simulink model "Model_Mk2"  (R2024a)
settings: Solver=VariableStepAuto  StartTime=startTime  StopTime=stopTime  FixedStep=1e-4  RelTol=1e-9  AbsTol=1e-9  EnableMultiTasking=on
model workspace (MAT data in the model file):
  Kset = [-2.00916512617e-14 -2.1396164685e-13 1645.65145003 1.10700309911e-13 0.064606154931 -1.15620600709 -2.35613942722e-12 1.21905689036 1.1835423475 0.0960813361903 -1.05646659933e-12 0.256355277786 ... (180 elements, 4x15x3)]
  MOI = [0.25  0.023  -0.0888; 0.023  0.5  0.097345; -0.0888  0.097345  0.5]
  betaInputDelay = 0.001
  discretize_interval = 0.0025
  g = 9.81
  gammaInputDelay = 0.001
  inputLimits = [-0.261799387799  0.261799387799; -0.261799387799  0.261799387799; 0  100; -0.1  0.1]
  l = 0.5
  m = 5
  q1 = [0.506236006596; 0.0473671727454; 0.176776695297]
  startTime = 0
  stopTime = 15
  tSegs = [0 7.5 15]
  t_set = [0 0.000750075007501 0.001500150015 0.0022502250225 0.00300030003 0.0037503750375 0.004500450045 0.00525052505251 0.00600060006001 0.00675067506751 0.00750075007501 0.00825082508251 ... (19999 elements, 1x19999)]
  throttleConsts = [71.0072; 0.0504; 67.9056]
  u_set = [-0.261799387799 0.261799387799 0 -0.1 -0.261799387799 0.261799387799 0 -0.1 -0.261799387799 0.261799387799 0 -0.1 ... (79996 elements, 4x19999)]
  x1 = [10; 5; 5; 0; 0; 0; 0.506236006596; 0.0473671727454; 0.176776695297; 0; 0; 0]
  x_set = [10 5 5 0 0 0 0.506236006596 0.0473671727454 0.176776695297 0 0 0 ... (239988 elements, 12x19999)]
undefined symbols (not defined in the file): DiscIntNeverNeededParam
libraries: matrix_library x2, sharedtransform x2, aerolibutil x1, vrlib x1
(part 2 of 2)

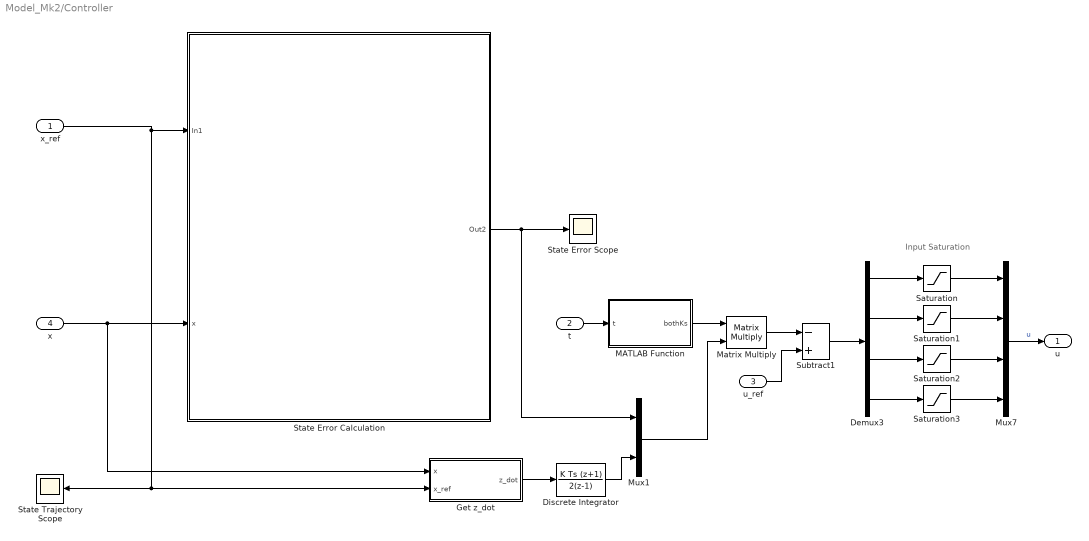
== system Model_Mk2/Controller ==
  note: Input Saturation
  x_ref : Inport
  t : Inport  Port=2
  u_ref : Inport  Port=3
  x : Inport  Port=4
  Demux3 : Demux
  Discrete Integrator : DiscreteIntegrator  IntegratorMethod=Integration: Trapezoidal  SampleTime=discretize_interval  ICPrevOutput=DiscIntNeverNeededParam  ICPrevScaledInput=DiscIntNeverNeededParam
  Get z_dot : MATLAB Function  TreatAsAtomicUnit=on
  MATLAB Function : MATLAB Function  TreatAsAtomicUnit=on
  Matrix Multiply : Product  Multiplication=Matrix(*)
  Mux1 : Mux  Inputs=2
  Mux7 : Mux
  Saturation : Saturate  UpperLimit=inputLimits(1, 2)  LowerLimit=inputLimits(1, 1)  LinearizeAsGain=off
  Saturation1 : Saturate  UpperLimit=inputLimits(2, 2)  LowerLimit=inputLimits(2, 1)  LinearizeAsGain=off
  Saturation2 : Saturate  UpperLimit=inputLimits(3, 2)  LowerLimit=inputLimits(3, 1)  LinearizeAsGain=off  ZeroCross=off
  Saturation3 : Saturate  UpperLimit=inputLimits(4, 2)  LowerLimit=inputLimits(4, 1)  LinearizeAsGain=off
  State Error Calculation : Subsystem
  State Error Scope : Scope
  State Trajectory Scope : Scope
  Subtract1 : Sum  Inputs=-+
  u : Outport
  wires:
  Saturation/1 -> Mux7/1
  Demux3/4 -> Saturation3/1
  Mux7/1 -> u/1  "u"
  Saturation1/1 -> Mux7/2
  Demux3/3 -> Saturation2/1
  Demux3/2 -> Saturation1/1
  Saturation2/1 -> Mux7/3
  Demux3/1 -> Saturation/1
  MATLAB Function/1(bothKs) -> Matrix Multiply/1
  u_ref/1 -> Subtract1/2
  Matrix Multiply/1 -> Subtract1/1
  Mux1/1 -> Matrix Multiply/2
  Subtract1/1 -> Demux3/1
  Get z_dot/1(z_dot) -> Discrete Integrator/1
  Saturation3/1 -> Mux7/4
  Discrete Integrator/1 -> Mux1/2
  t/1 -> MATLAB Function/1(t)
  x_ref/1 -> Get z_dot/2(x_ref), State Trajectory Scope/1, State Error Calculation/1(In1)
  x/1 -> State Error Calculation/2(x), Get z_dot/1(x)
  State Error Calculation/1(Out2) -> Mux1/1, State Error Scope/1

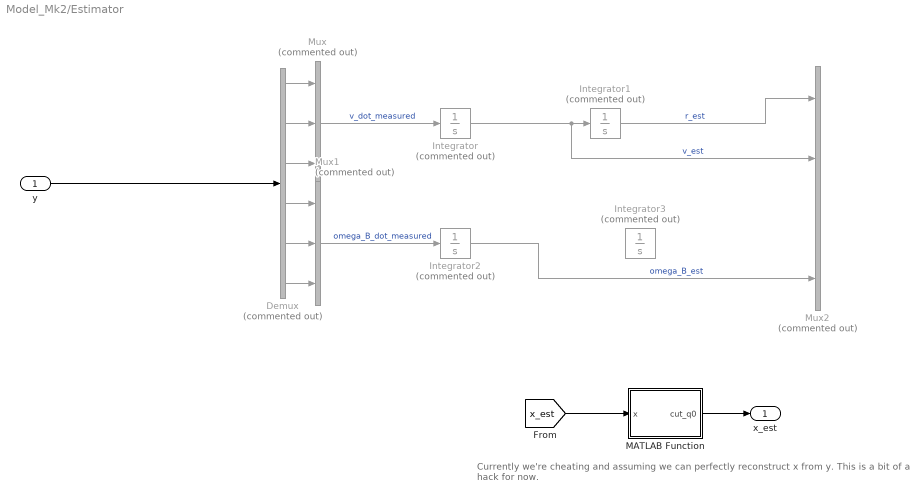
== system Model_Mk2/Estimator ==
  note: Currently we're cheating and assuming we can perfectly reconstruct x from y. This is a bit of a hack for now.
  y : Inport
  Demux : Demux  Commented=on  Outputs=6
  Integrator : Integrator  Commented=on  InitialCondition=x1(4:6)
  Integrator1 : Integrator  Commented=on  InitialCondition=x1(1:3)
  Integrator2 : Integrator  Commented=on  InitialCondition=x1(4:6)
  Integrator3 : Integrator  Commented=on  InitialCondition=x1(1:3)
  MATLAB Function : MATLAB Function  TreatAsAtomicUnit=on
  Mux : Mux  Commented=on  Inputs=3
  Mux1 : Mux  Commented=on  Inputs=3
  Mux2 : Mux  Commented=on
  x_est : Outport
  wires:
  Demux/1 -> Mux/1
  Demux/2 -> Mux/2
  Demux/3 -> Mux/3
  Demux/6 -> Mux1/3
  Demux/5 -> Mux1/2
  Demux/4 -> Mux1/1
  Mux/1 -> Integrator/1  "v_dot_measured"
  Integrator/1 -> Mux2/2, Integrator1/1  "v_est"
  Integrator1/1 -> Mux2/1  "r_est"
  Integrator2/1 -> Mux2/4  "omega_B_est"
  Mux1/1 -> Integrator2/1  "omega_B_dot_measured"
  y/1 -> Demux/1
  MATLAB Function/1(cut_q0) -> x_est/1
  [x_est] -> MATLAB Function/1(x)

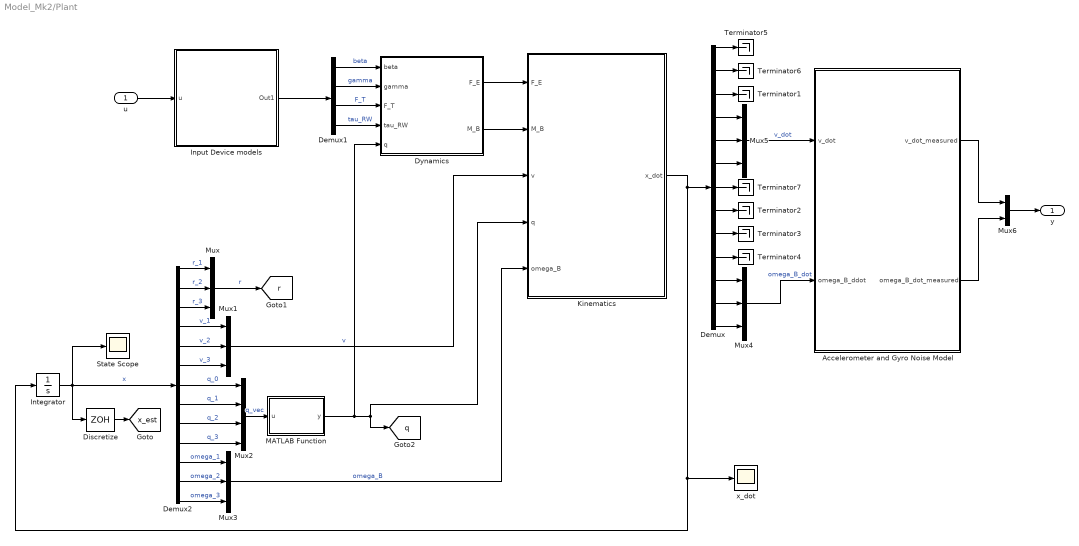
== system Model_Mk2/Plant ==
  u : Inport
  Accelerometer and Gyro Noise Model : Subsystem
  Demux : Demux  Outputs=13
  Demux1 : Demux
  Demux2 : Demux  Outputs=13
  Discretize : ZeroOrderHold  SampleTime=-1
  Dynamics : Subsystem
  Input Device models : Subsystem
  Integrator : Integrator  InitialCondition=[x1(1:6); sqrt(1-q1(1)^2-q1(2)^2-q1(3)^2); x1(7:end)]
  Kinematics : Subsystem
  MATLAB Function : MATLAB Function  TreatAsAtomicUnit=on
  Mux{,1,3..5} (5 alike) : Mux  Inputs=3
  Mux2 : Mux
  Mux6 : Mux  Inputs=2
  State Scope : Scope
  Terminator{1..7} (7 alike) : Terminator
  x_dot : Scope
  y : Outport
  tag scope: q=global, r=global, x_est=global
  wires:
  Dynamics/1(F_E) -> Kinematics/1(F_E)
  Dynamics/2(M_B) -> Kinematics/2(M_B)
  Demux1/1 -> Dynamics/1(beta)  "beta"
  Demux1/2 -> Dynamics/2(gamma)  "gamma"
  Demux1/3 -> Dynamics/3(F_T)  "F_T"
  Demux1/4 -> Dynamics/4(tau_RW)  "tau_RW"
  Integrator/1 -> State Scope/1, Demux2/1, Discretize/1  "x"
  Demux2/1 -> Mux/1  "r_1"
  Demux2/2 -> Mux/2  "r_2"
  Demux2/3 -> Mux/3  "r_3"
  Mux/1 -> [r]  "r"
  Demux2/4 -> Mux1/1  "v_1"
  Demux2/5 -> Mux1/2  "v_2"
  Demux2/6 -> Mux1/3  "v_3"
  Mux1/1 -> Kinematics/3(v)  "v"
  Demux2/8 -> Mux2/2  "q_1"
  Demux2/9 -> Mux2/3  "q_2"
  Demux2/13 -> Mux3/3  "omega_3"
  Demux2/12 -> Mux3/2  "omega_2"
  Demux2/11 -> Mux3/1  "omega_1"
  Mux2/1 -> MATLAB Function/1(u)  "q_vec"
  Mux3/1 -> Kinematics/5(omega_B)  "omega_B"
  Kinematics/1(x_dot) -> x_dot/1, Integrator/1, Demux/1
  Demux/11 -> Mux4/1
  Demux/12 -> Mux4/2
  Demux/13 -> Mux4/3
  Demux/5 -> Mux5/2
  Demux/4 -> Mux5/1
  Demux/3 -> Terminator1/1
  Mux5/1 -> Accelerometer and Gyro Noise Model/1(v_dot)  "v_dot"
  Mux4/1 -> Accelerometer and Gyro Noise Model/2(omega_B_ddot)  "omega_B_dot"
  Demux/8 -> Terminator2/1
  Demux/9 -> Terminator3/1
  Demux/10 -> Terminator4/1
  Accelerometer and Gyro Noise Model/1(v_dot_measured) -> Mux6/1
  Accelerometer and Gyro Noise Model/2(omega_B_dot_measured) -> Mux6/2
  Mux6/1 -> y/1
  Demux/1 -> Terminator5/1
  Demux/2 -> Terminator6/1
  Demux/6 -> Mux5/3
  Input Device models/1(Out1) -> Demux1/1
  u/1 -> Input Device models/1(u)
  Demux2/10 -> Mux2/4  "q_3"
  Demux2/7 -> Mux2/1  "q_0"
  Demux/7 -> Terminator7/1
  MATLAB Function/1(y) -> Dynamics/5(q), Kinematics/4(q), [q]
  Discretize/1 -> [x_est]

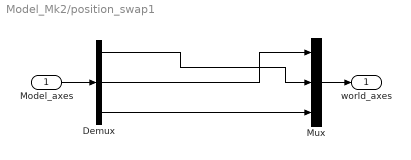
== system Model_Mk2/position_swap1 ==
  Model_axes : Inport
  Demux : Demux  Outputs=3
  Mux : Mux  Inputs=3
  world_axes : Outport
  wires:
  Mux/1 -> world_axes/1
  Model_axes/1 -> Demux/1
  Demux/2 -> Mux/1
  Demux/1 -> Mux/2
  Demux/3 -> Mux/3

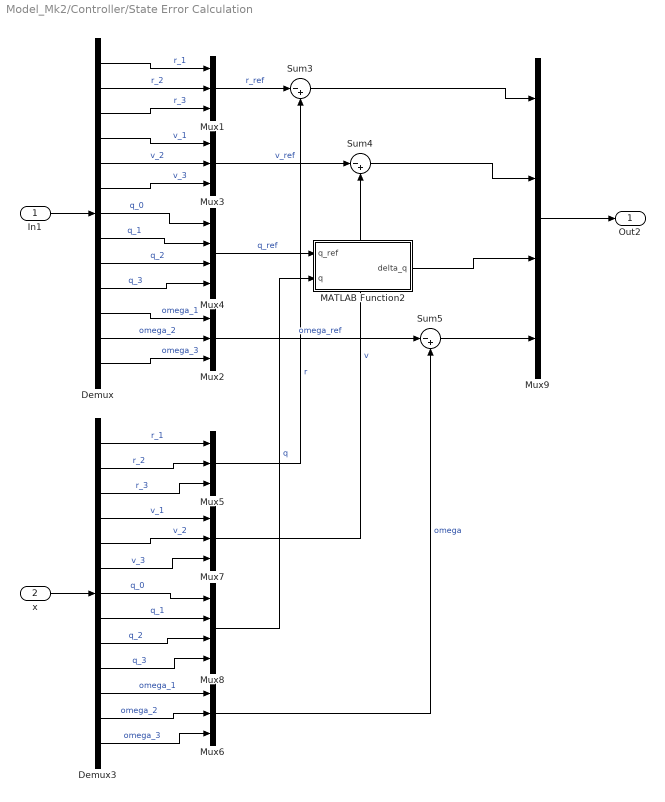
== system Model_Mk2/Controller/State Error Calculation ==
  In1 : Inport
  x : Inport  Port=2
  Demux : Demux  Outputs=13
  Demux3 : Demux  Outputs=13
  MATLAB Function2 : MATLAB Function  TreatAsAtomicUnit=on
  Mux{1..3,5..7} (6 alike) : Mux  Inputs=3
  Mux4 : Mux
  Mux8 : Mux
  Mux9 : Mux
  Sum3 : Sum  Inputs=|-+
  Sum4 : Sum  Inputs=|-+
  Sum5 : Sum  Inputs=|-+
  Out2 : Outport
  wires:
  In1/1 -> Demux/1
  Demux/1 -> Mux1/1  "r_1"
  Demux/2 -> Mux1/2  "r_2"
  Demux/3 -> Mux1/3  "r_3"
  Demux/12 -> Mux2/2  "omega_2"
  Demux/11 -> Mux2/1  "omega_1"
  Demux/13 -> Mux2/3  "omega_3"
  Demux/4 -> Mux3/1  "v_1"
  Demux/5 -> Mux3/2  "v_2"
  Demux/6 -> Mux3/3  "v_3"
  Demux/8 -> Mux4/2  "q_1"
  Demux/9 -> Mux4/3  "q_2"
  Demux/10 -> Mux4/4  "q_3"
  Demux/7 -> Mux4/1  "q_0"
  Demux3/11 -> Mux6/1  "omega_1"
  Demux3/2 -> Mux5/2  "r_2"
  Demux3/7 -> Mux8/1  "q_0"
  Demux3/5 -> Mux7/2  "v_2"
  Demux3/9 -> Mux8/3  "q_2"
  Demux3/12 -> Mux6/2  "omega_2"
  Demux3/10 -> Mux8/4  "q_3"
  Demux3/8 -> Mux8/2  "q_1"
  Demux3/4 -> Mux7/1  "v_1"
  Demux3/3 -> Mux5/3  "r_3"
  x/1 -> Demux3/1
  Demux3/6 -> Mux7/3  "v_3"
  Demux3/1 -> Mux5/1  "r_1"
  Demux3/13 -> Mux6/3  "omega_3"
  Mux5/1 -> Sum3/2  "r"
  Mux1/1 -> Sum3/1  "r_ref"
  Mux3/1 -> Sum4/1  "v_ref"
  Mux7/1 -> Sum4/2  "v"
  Mux2/1 -> Sum5/1  "omega_ref"
  Mux6/1 -> Sum5/2  "omega"
  Mux4/1 -> MATLAB Function2/1(q_ref)  "q_ref"
  Mux8/1 -> MATLAB Function2/2(q)  "q"
  Sum5/1 -> Mux9/4
  Sum3/1 -> Mux9/1
  Sum4/1 -> Mux9/2
  MATLAB Function2/1(delta_q) -> Mux9/3
  Mux9/1 -> Out2/1

== system Model_Mk2/Plant/Accelerometer and Gyro Noise Model ==
  v_dot : Inport
  omega_B_ddot : Inport  Port=2
  v_dot_measured : Outport
  omega_B_dot_measured : Outport  Port=2
  wires:
  v_dot/1 -> v_dot_measured/1
  omega_B_ddot/1 -> omega_B_dot_measured/1

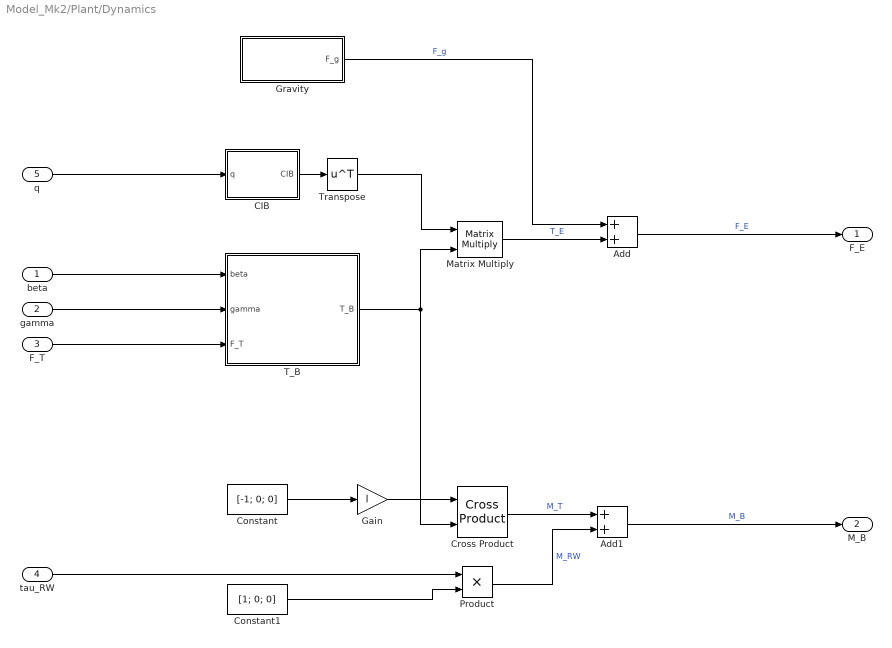
== system Model_Mk2/Plant/Dynamics ==
  beta : Inport
  gamma : Inport  Port=2
  F_T : Inport  Port=3
  tau_RW : Inport  Port=4
  q : Inport  Port=5
  Add : Sum
  Add1 : Sum
  CIB : MATLAB Function  TreatAsAtomicUnit=on
  Constant : Constant  Value=[-1; 0; 0]
  Constant1 : Constant  Value=[1; 0; 0]
  Cross Product : matrix_library/Cross Product
  Gain : Gain  Gain=l
  Gravity : Subsystem
  Matrix Multiply : Product  Multiplication=Matrix(*)
  Product : Product
  T_B : Subsystem
  Transpose : Math  Operator=transpose
  F_E : Outport
  M_B : Outport  Port=2
  wires:
  beta/1 -> T_B/1(beta)
  gamma/1 -> T_B/2(gamma)
  F_T/1 -> T_B/3(F_T)
  q/1 -> CIB/1(q)
  T_B/1(T_B) -> Cross Product/2, Matrix Multiply/2
  Matrix Multiply/1 -> Add/2  "T_E"
  Gravity/1(F_g) -> Add/1  "F_g"
  Gain/1 -> Cross Product/1
  Constant/1 -> Gain/1
  Constant1/1 -> Product/2
  tau_RW/1 -> Product/1
  Product/1 -> Add1/2  "M_RW"
  Cross Product/1 -> Add1/1  "M_T"
  Add1/1 -> M_B/1  "M_B"
  Add/1 -> F_E/1  "F_E"
  CIB/1(CIB) -> Transpose/1
  Transpose/1 -> Matrix Multiply/1

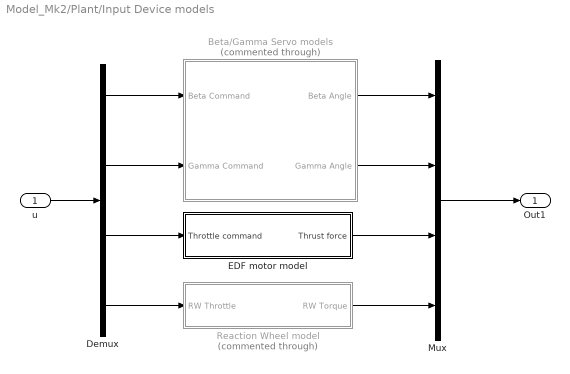
== system Model_Mk2/Plant/Input Device models ==
  u : Inport
  Beta/Gamma Servo models : Subsystem  Commented=through
  Demux : Demux
  EDF motor model : Subsystem
  Mux : Mux
  Reaction Wheel model : Subsystem  Commented=through
  Out1 : Outport
  wires:
  u/1 -> Demux/1
  Demux/1 -> Beta/Gamma Servo models/1(Beta Command)
  Demux/2 -> Beta/Gamma Servo models/2(Gamma Command)
  Demux/3 -> EDF motor model/1(Throttle command)
  Demux/4 -> Reaction Wheel model/1(RW Throttle)
  Mux/1 -> Out1/1
  Beta/Gamma Servo models/1(Beta Angle) -> Mux/1
  Beta/Gamma Servo models/2(Gamma Angle) -> Mux/2
  EDF motor model/1(Thrust force) -> Mux/3
  Reaction Wheel model/1(RW Torque) -> Mux/4

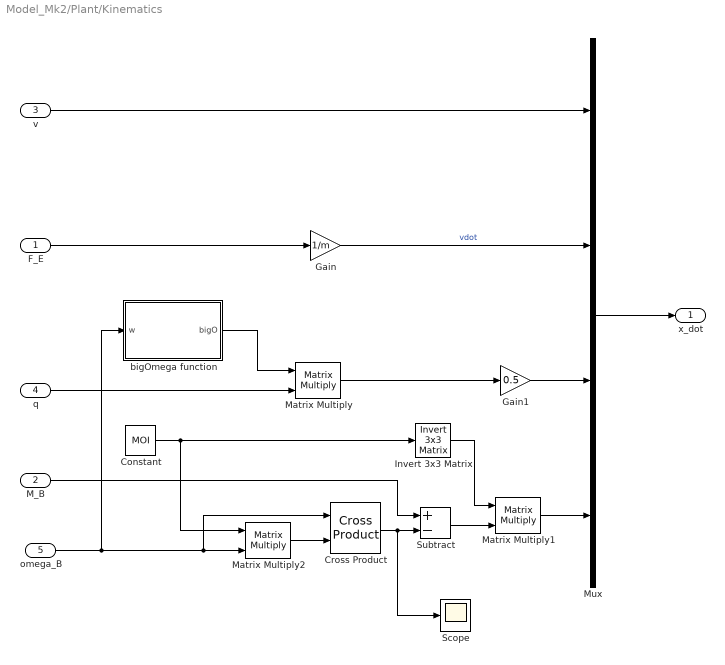
== system Model_Mk2/Plant/Kinematics ==
  F_E : Inport
  M_B : Inport  Port=2
  v : Inport  Port=3
  q : Inport  Port=4
  omega_B : Inport  Port=5
  Constant : Constant  Value=MOI
  Cross Product : matrix_library/Cross Product
  Gain : Gain  Gain=1/m
  Gain1 : Gain  Gain=0.5
  Invert 3x3 Matrix : aerolibutil/Invert  3x3 Matrix
  Matrix Multiply : Product  Multiplication=Matrix(*)
  Matrix Multiply1 : Product  Multiplication=Matrix(*)
  Matrix Multiply2 : Product  Multiplication=Matrix(*)
  Mux : Mux
  Scope : Scope
  Subtract : Sum  Inputs=+-
  bigOmega function : MATLAB Function  TreatAsAtomicUnit=on
  x_dot : Outport
  wires:
  q/1 -> Matrix Multiply/2
  Matrix Multiply2/1 -> Cross Product/2
  bigOmega function/1(bigO) -> Matrix Multiply/1
  Matrix Multiply/1 -> Gain1/1
  Constant/1 -> Invert 3x3 Matrix/1, Matrix Multiply2/1
  F_E/1 -> Gain/1
  omega_B/1 -> Cross Product/1, Matrix Multiply2/2, bigOmega function/1(w)
  Gain1/1 -> Mux/3
  M_B/1 -> Subtract/1
  Cross Product/1 -> Scope/1, Subtract/2
  Invert 3x3 Matrix/1 -> Matrix Multiply1/1
  Subtract/1 -> Matrix Multiply1/2
  v/1 -> Mux/1
  Gain/1 -> Mux/2  "vdot"
  Matrix Multiply1/1 -> Mux/4
  Mux/1 -> x_dot/1

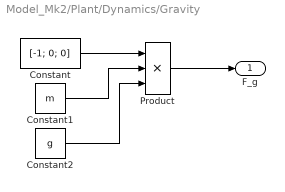
== system Model_Mk2/Plant/Dynamics/Gravity ==
  Constant : Constant  Value=[-1; 0; 0]
  Constant1 : Constant  Value=m
  Constant2 : Constant  Value=g
  Product : Product  Inputs=3
  F_g : Outport
  wires:
  Constant/1 -> Product/1
  Constant2/1 -> Product/3
  Constant1/1 -> Product/2
  Product/1 -> F_g/1

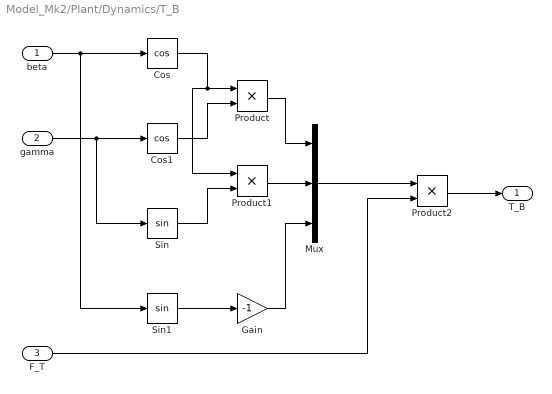
== system Model_Mk2/Plant/Dynamics/T_B ==
  beta : Inport
  gamma : Inport  Port=2
  F_T : Inport  Port=3
  Cos : Trigonometry  Operator=cos
  Cos1 : Trigonometry  Operator=cos
  Gain : Gain  Gain=-1
  Mux : Mux  Inputs=3
  Product : Product
  Product1 : Product
  Product2 : Product
  Sin : Trigonometry
  Sin1 : Trigonometry
  T_B : Outport
  wires:
  Cos/1 -> Product/1, Product1/1
  Cos1/1 -> Product/2
  beta/1 -> Sin1/1, Cos/1
  gamma/1 -> Sin/1, Cos1/1
  Sin/1 -> Product1/2
  Sin1/1 -> Gain/1
  Gain/1 -> Mux/3
  Product1/1 -> Mux/2
  Product/1 -> Mux/1
  Mux/1 -> Product2/1
  F_T/1 -> Product2/2
  Product2/1 -> T_B/1

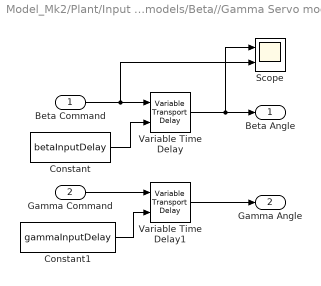
== system Model_Mk2/Plant/Input Device models/Beta//Gamma Servo models ==
  Beta Command : Inport
  Gamma Command : Inport  Port=2
  Constant : Constant  Value=betaInputDelay
  Constant1 : Constant  Value=gammaInputDelay
  Scope : Scope  NumInputPorts=2
  Variable Time Delay : VariableTransportDelay  MaximumDelay=10
  Variable Time Delay1 : VariableTransportDelay  MaximumDelay=10
  Beta Angle : Outport
  Gamma Angle : Outport  Port=2
  wires:
  Beta Command/1 -> Variable Time Delay/1, Scope/2
  Variable Time Delay/1 -> Beta Angle/1, Scope/1
  Variable Time Delay1/1 -> Gamma Angle/1
  Gamma Command/1 -> Variable Time Delay1/1
  Constant/1 -> Variable Time Delay/2
  Constant1/1 -> Variable Time Delay1/2

== system Model_Mk2/Plant/Input Device models/EDF motor model ==
  Throttle command : Inport
  Constant : Constant  Value=throttleConsts
  MATLAB Function : MATLAB Function  TreatAsAtomicUnit=on
  Thrust force : Outport
  wires:
  Throttle command/1 -> MATLAB Function/1(throttle)
  MATLAB Function/1(F_T) -> Thrust force/1
  Constant/1 -> MATLAB Function/2(throttleConsts)

== system Model_Mk2/Plant/Input Device models/Reaction Wheel model ==
  RW Throttle : Inport
  RW Torque : Outport
  wires:
  RW Throttle/1 -> RW Torque/1

== matlab function Model_Mk2/Controller/Get z_dot ==
  data: x input; z_dot output; x_ref input
function z_dot = getZDot(x, x_ref)
C = [eye(3), zeros(3, length(x) - 3)];
z_dot = C*x - x_ref(1:3);

== matlab function Model_Mk2/Get State Trajectory ==
  data: t input; x_ref output; x_set parameter; t_set parameter
function x_ref = get_trajectory(t, x_set, t_set)
    x_ref = zeros(size(x_set, 1), 1);
    for i = 1:size(x_ref, 1)
        x_ref(i) = interp1(t_set, x_set(i, :), t);
    end
end

== matlab function Model_Mk2/Controller/MATLAB Function ==
  data: t input; bothKs output; Kset parameter; tSegs parameter
function bothKs = fcn(t, Kset, tSegs)
currentIndex = -1;
for i = 1:length(tSegs)
    if (i ~= 1) && (t <= tSegs(i))
        currentIndex = i-1;
        break;
    end
end

bothKs = Kset(:, :, currentIndex);

== matlab function Model_Mk2/Plant/Input Device models/EDF motor model/MATLAB Function ==
  data: throttle input; F_T output; throttleConsts input
% function F_T = fcn(throttle)
% F_T = polyval(flip(throttleCoeffs), throttle - 50);

function F_T = fcn(throttle, throttleConsts)
F_T = throttleConsts(1) ./ (1 + exp(-throttleConsts(2)*(throttle-throttleConsts(3))));

== matlab function Model_Mk2/Estimator/MATLAB Function ==
  data: x input; cut_q0 output
function cut_q0 = fcn(x)
cut_q0 = x([1:6, 8:end]);

== matlab function Model_Mk2/Get Input Trajectory ==
  data: t input; u_ref output; u_set parameter; t_set parameter
function u_ref = get_trajectory(t, u_set, t_set)
    u_ref = zeros(size(u_set, 1), 1);
    for i = 1:size(u_set, 1)
        u_ref(i) = interp1(t_set, u_set(i, :), t);
    end
end

== matlab function Model_Mk2/Plant/Dynamics/CIB ==
  data: q input; CIB output
function CIB = quatRot(q)
    q0 = q(1);
    q1 = q(2);
    q2 = q(3);
    q3 = q(4);
    CIB = [1-2*(q2^2 + q3^2), 2*(q1*q2 + q0*q3), 2*(q1*q3 - q0*q2);
        2*(q1*q2 - q0*q3), 1-2*(q1^2 + q3^2), 2*(q2*q3 + q0*q1);
        2*(q1*q3 + q0*q2), 2*(q2*q3 - q0*q1), 1-2*(q1^2 + q2^2)];
end

== matlab function Model_Mk2/Plant/MATLAB Function ==
  data: u input; y output
function y = normalize(u)
y = u / norm(u, 2);

== matlab function Model_Mk2/Controller/State Error Calculation/MATLAB Function2 ==
  data: q_ref input; q input; delta_q output
function delta_q = get_delta_q(q_ref,q)
% difference of quaternions in SO(3) [ q - q_ref  ~> (q_ref*) prod q]
% scalar first convention
LT = [q_ref(1) q_ref(2) q_ref(3) q_ref(4);
    -q_ref(2) q_ref(1) q_ref(4) -q_ref(3);
    -q_ref(3) -q_ref(4) q_ref(1) q_ref(2);
    -q_ref(4) q_ref(3) -q_ref(2) q_ref(1)];
% multiplication by conjugate
delta_q = LT * q;
end

== matlab function Model_Mk2/Plant/Kinematics/bigOmega function ==
  data: w input size=[3 1]; bigO output
function bigO = bigOmega(w)
bigO = [0    -w(1) -w(2) -w(3);
        w(1)  0     w(3) -w(2);
        w(2) -w(3)  0     w(1);
        w(3)  w(2) -w(1)  0  ];
end
